simulink model "doc_filtercutoffs"  (Simulink 6.0)
settings: Solver=ode45  StartTime=0.0  StopTime=10.0  RelTol=1e-3
undefined symbols (not defined in the file): slcm
libraries: commanapbnd2 x2
settings Model: Creator=mmclerno  LastModifiedBy=agaltman  ProdHWDeviceType=Specified
settings DataIOCC: SignalLoggingName=logsOut
settings OptimizationCC: BlockReduction=off  BooleanDataType=off  MultiInstanced=off
settings FormatCC: IgnoreBidirectionalLines=off
settings HardwareCC: ProdHWDeviceType=Specified
settings CodeAppCC: FileBanners=off  CustomSymbols=off  MangleLength=5
settings GRTTargetCC: TargetFcnLib=iso_c_tmw.mat  IsERTTarget=off

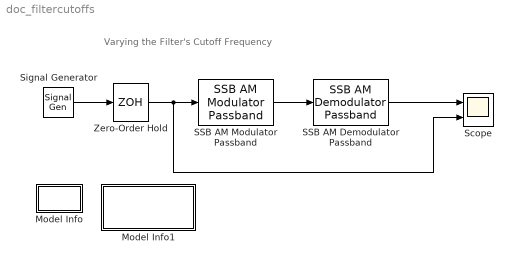
== system doc_filtercutoffs ==
  note: Varying the Filter's Cutoff Frequency
  Model Info : Subsystem  LoadFcn=slcm LoadBlock;  InitFcn=slcm('UpdateAllCMBlocksInThisModelInit')  mask(CMBlock){InitialSaveTempField=, InitialBlockCM=none, BlockCM=none, Frame=on, SaveTempField=, DisplayStringWithTags=Info, MaskDisplayString=Info, HorizontalTextAlignment=Center, LeftAlignmentValue=0.5, SourceBlockDiagram=doc_filtercutoffs, TagMaxNumber=20, CMTag1=, CMTag2=, CMTag3=, CMTag4=, CMTag5=, CMTag6=, CMTag7=, CMTag8=, CMTag9=, CMTag10=, CMTag11=, CMTag12=, CMTag13=, CMTag14=, CMTag15=, CMTag16=, CMTag17=, CMTag18=, CMTag19=, CMTag20=}
      mask help: This block allows revision control information to be displayed within the model.
      settings: CopyFcn=slcm CopyBlock;  DeleteFcn=slcm Cancel;  PostSaveFcn=slcm('UpdateAllCMBlocksInThisModel')  NameChangeFcn=slcm Rename;  OpenFcn=commdemohelp;
      mask Display: text(str2num(LeftAlignmentValue), 0.5, MaskDisplayString, 'HorizontalAlignment', HorizontalTextAlignment)
  Model Info1 : Subsystem  LoadFcn=slcm LoadBlock;  InitFcn=slcm('UpdateAllCMBlocksInThisModelInit')  mask(CMBlock){InitialSaveTempField=, InitialBlockCM=none, BlockCM=none, Frame=on, SaveTempField=, DisplayStringWithTags=Info, MaskDisplayString=Info, HorizontalTextAlignment=Center, LeftAlignmentValue=0.5, SourceBlockDiagram=doc_filtercutoffs, TagMaxNumber=20, CMTag1=, CMTag2=, CMTag3=, CMTag4=, CMTag5=, CMTag6=, CMTag7=, CMTag8=, CMTag9=, CMTag10=, CMTag11=, CMTag12=, CMTag13=, CMTag14=, CMTag15=, CMTag16=, CMTag17=, CMTag18=, CMTag19=, CMTag20=}
      mask help: This block allows revision control information to be displayed within the model.
      settings: CopyFcn=slcm CopyBlock;  DeleteFcn=slcm Cancel;  PostSaveFcn=slcm('UpdateAllCMBlocksInThisModel')  NameChangeFcn=slcm Rename;  OpenFcn=[num,den] = butter(2,25*.01);
      mask Display: text(str2num(LeftAlignmentValue), 0.5, 'Double-click to\npreload data', 'HorizontalAlignment', HorizontalTextAlignment)
  SSB AM Demodulator Passband : commanapbnd2/SSB AM Demodulator Passband  Fc=25  num=num  den=den  Ph=0  ts=.01
  SSB AM Modulator Passband : commanapbnd2/SSB AM Modulator Passband  Fc=25  Ph=0  ban=10  dly=.1  ts=.01  sd=Upper
  Scope : Scope  NumInputPorts=2
      settings: YMin=-5~-5  YMax=5~5
  Signal Generator : SignalGenerator  WaveForm=sawtooth  Amplitude=4  Frequency=.3
  Zero-Order Hold : ZeroOrderHold  SampleTime=.01
  wires:
  Zero-Order Hold/1 -> SSB AM Modulator Passband/1, Scope/2
  Signal Generator/1 -> Zero-Order Hold/1
  SSB AM Modulator Passband/1 -> SSB AM Demodulator Passband/1
  SSB AM Demodulator Passband/1 -> Scope/1

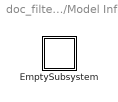
== system doc_filtercutoffs/Model Info ==
  EmptySubsystem : Subsystem

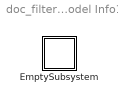
== system doc_filtercutoffs/Model Info1 ==
  EmptySubsystem : Subsystem

== system doc_filtercutoffs/Model Info/EmptySubsystem ==

== system doc_filtercutoffs/Model Info1/EmptySubsystem ==
